simulink model "LMS_MODEL"  (R2015b)
settings: Solver=VariableStepAuto  StartTime=0.0  StopTime=30.0  RelTol=1e-3
libraries: dspsrcs4 x2, dspadpt3 x1, dspsnks4 x1
settings Model: Creator=RAGHAVA  LastModifiedBy=Pranshu

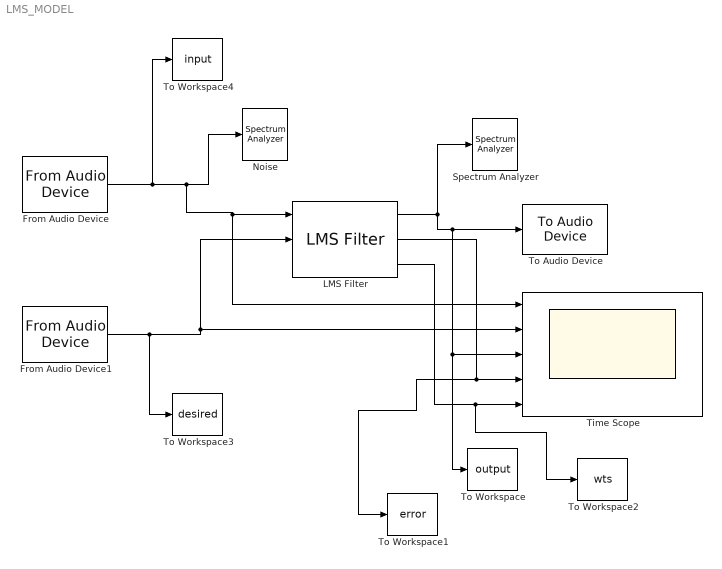
== system LMS_MODEL ==
  From Audio Device : dspsrcs4/From Audio Device  deviceName=Default  numChannels=1  sampleRate=44100  deviceDatatype=Determine from output data type  autoBufferSize=on  bufferSize=4096  queueDuration=1.0  frameSize=1024  outputDatatype=single  defaultInputChannelMapping=on  inputChannelMapping=1:2  outputNumOverrunSamples=off  OutputFrames=off
  From Audio Device1 : dspsrcs4/From Audio Device  deviceName=Microphone (Conexant SmartAudio HD)  numChannels=1  sampleRate=44100  deviceDatatype=Determine from output data type  autoBufferSize=on  bufferSize=4096  queueDuration=1.0  frameSize=1024  outputDatatype=single  defaultInputChannelMapping=on  inputChannelMapping=1:2  outputNumOverrunSamples=off  OutputFrames=off
  LMS Filter : dspadpt3/LMS Filter  Algo=Normalized LMS  L=30  stepflag=Dialog  mu=0.1  leakage=1.0  ic=0  Adapt=off  resetflag=Non-zero sample  weights=on  firstCoeffMode=Specify word length  firstCoeffWordLength=32  firstCoeffFracLength=15  secondCoeffMode=User-defined  secondCoeffWordLength=2  secondCoeffFracLength=15  accum2Mode=User-defined  accum2FracLength=20  prodOutputMode=Slope and bias scaling  prodOutputWordLength=32  prodOutputFracLength=20  prodOutput2Mode=User-defined  prodOutput2FracLength=20  prodOutput3Mode=User-defined  prodOutput3FracLength=20  prodOutput4Mode=User-defined  prodOutput4FracLength=20  quotientMode=User-defined  quotientFracLength=20  roundingMode=Floor  overflowMode=off  addnparflag=off
  Noise : SpectrumAnalyzer
  Spectrum Analyzer : SpectrumAnalyzer
  Time Scope : Scope  NumInputPorts=5
  To Audio Device : dspsnks4/To Audio Device  deviceName=Default  inheritSampleRate=on  sampleRate=44100  deviceDatatype=Determine from input data type  autoBufferSize=on  bufferSize=4096  queueDuration=1.0  defaultOutputChannelMapping=on  outputChannelMapping=1:2  outputNumUnderrunSamples=off
  To Workspace : ToWorkspace  VariableName=output  SampleTime=-1
      settings: Save2DSignal=2-D array (concatenate along first dimension)
  To Workspace1 : ToWorkspace  VariableName=error  SampleTime=-1
      settings: Save2DSignal=2-D array (concatenate along first dimension)
  To Workspace2 : ToWorkspace  VariableName=wts  SampleTime=-1
      settings: Save2DSignal=2-D array (concatenate along first dimension)
  To Workspace3 : ToWorkspace  VariableName=desired  SampleTime=-1
      settings: Save2DSignal=2-D array (concatenate along first dimension)
  To Workspace4 : ToWorkspace  VariableName=input  SampleTime=-1
      settings: Save2DSignal=2-D array (concatenate along first dimension)
  wires:
  LMS Filter/1 -> To Audio Device/1, Time Scope/3, To Workspace/1, Spectrum Analyzer/1
  From Audio Device1/1 -> To Workspace3/1, Time Scope/2, LMS Filter/2
  LMS Filter/2 -> To Workspace1/1, Time Scope/4
  LMS Filter/3 -> To Workspace2/1, Time Scope/5
  From Audio Device/1 -> To Workspace4/1, Noise/1, Time Scope/1, LMS Filter/1
